simulink model "startOLAE"  (R2021a)
settings: Solver=VariableStepAuto  StartTime=0.0  StopTime=10.0  RelTol=1e-3
libraries: sharedutil x2, dspmtrx3 x1, aerolibutil x1
settings Model: Creator=noraw  LastModifiedBy=noraw

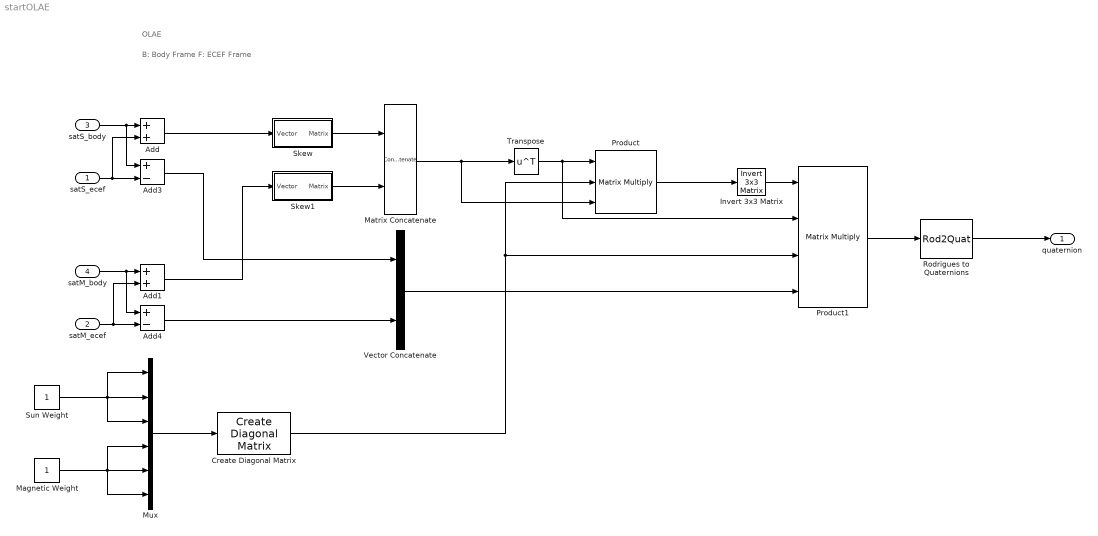
== system startOLAE ==
  note: OLAE
  note: B: Body Frame
      | F: ECEF Frame
  satS_ecef : Inport  PortDimensions=3
  satM_ecef : Inport  Port=2  PortDimensions=3
  satS_body : Inport  Port=3  PortDimensions=3
  satM_body : Inport  Port=4  PortDimensions=3
  Add : Sum
  Add1 : Sum
  Add3 : Sum  Inputs=+-
  Add4 : Sum  Inputs=+-
  Create Diagonal Matrix : dspmtrx3/Create Diagonal Matrix
      settings: SourceProductBaseCode=DS
  Invert 3x3 Matrix : aerolibutil/Invert  3x3 Matrix
  Magnetic Weight : Constant
  Matrix Concatenate : Concatenate  Mode=Multidimensional array
  Mux : Mux  Inputs=6
  Product : Product  Inputs=3  Multiplication=Matrix(*)
  Product1 : Product  Inputs=4  Multiplication=Matrix(*)
  Rodrigues to Quaternions : Rod2Quat
  Skew : Subsystem
  Skew1 : Subsystem
  Sun Weight : Constant
  Transpose : Math  Operator=transpose  SaturateOnIntegerOverflow=on
  Vector Concatenate : Concatenate
  quaternion : Outport
  wires:
  Matrix Concatenate/1 -> Product/3, Transpose/1
  Product/1 -> Invert 3x3 Matrix/1
  Sun Weight/1 -> Mux/1, Mux/2, Mux/3
  Invert 3x3 Matrix/1 -> Product1/1
  Product1/1 -> Rodrigues to Quaternions/1
  Transpose/1 -> Product1/2, Product/1
  Skew/1(Matrix) -> Matrix Concatenate/1
  Magnetic Weight/1 -> Mux/4, Mux/5, Mux/6
  Skew1/1(Matrix) -> Matrix Concatenate/2
  Create Diagonal Matrix/1 -> Product/2, Product1/3
  Mux/1 -> Create Diagonal Matrix/1
  satS_body/1 -> Add3/1, Add/1
  Add1/1 -> Skew1/1(Vector)
  satM_ecef/1 -> Add1/2, Add4/2
  Add/1 -> Skew/1(Vector)
  satM_body/1 -> Add4/1, Add1/1
  Add4/1 -> Vector Concatenate/2
  Rodrigues to Quaternions/1 -> quaternion/1
  Add3/1 -> Vector Concatenate/1
  satS_ecef/1 -> Add/2, Add3/2
  Vector Concatenate/1 -> Product1/4

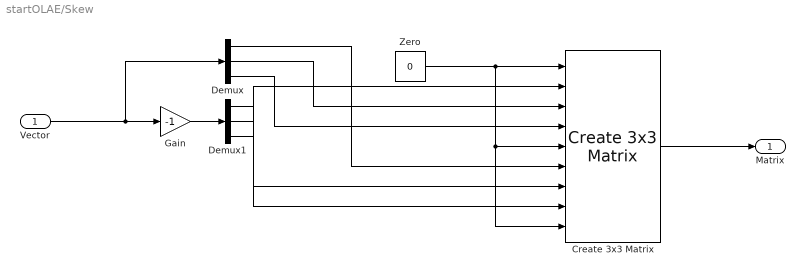
== system startOLAE/Skew ==
  Vector : Inport
  Create 3x3 Matrix : sharedutil/Create 3x3 Matrix  aMode=aMode
      settings: SourceProductBaseCode=AE,PW,MT,UV,VE,VP
  Demux : Demux  Outputs=3
  Demux1 : Demux  Outputs=3
  Gain : Gain  Gain=-1
  Zero : Constant  Value=0  OutDataTypeStr=Inherit: Inherit via back propagation
  Matrix : Outport
  wires:
  Gain/1 -> Demux1/1
  Demux/1 -> Create 3x3 Matrix/6
  Demux1/2 -> Create 3x3 Matrix/7
  Vector/1 -> Gain/1, Demux/1
  Demux1/1 -> Create 3x3 Matrix/8
  Demux1/3 -> Create 3x3 Matrix/2
  Zero/1 -> Create 3x3 Matrix/9, Create 3x3 Matrix/5, Create 3x3 Matrix/1
  Demux/3 -> Create 3x3 Matrix/4
  Demux/2 -> Create 3x3 Matrix/3
  Create 3x3 Matrix/1 -> Matrix/1

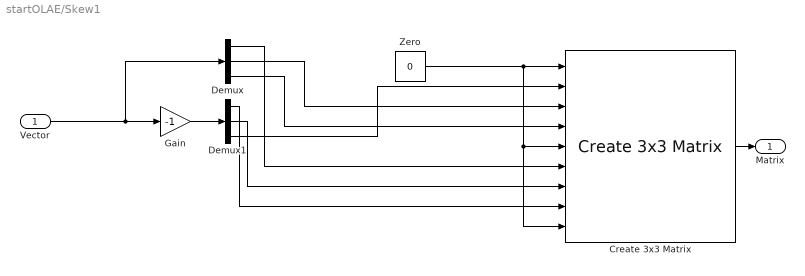
== system startOLAE/Skew1 ==
  Vector : Inport
  Create 3x3 Matrix : sharedutil/Create 3x3 Matrix  aMode=aMode
      settings: SourceProductBaseCode=AE,PW,MT,UV,VE,VP
  Demux : Demux  Outputs=3
  Demux1 : Demux  Outputs=3
  Gain : Gain  Gain=-1
  Zero : Constant  Value=0  OutDataTypeStr=Inherit: Inherit via back propagation
  Matrix : Outport
  wires:
  Gain/1 -> Demux1/1
  Demux/1 -> Create 3x3 Matrix/6
  Demux1/2 -> Create 3x3 Matrix/7
  Vector/1 -> Gain/1, Demux/1
  Demux1/1 -> Create 3x3 Matrix/8
  Demux1/3 -> Create 3x3 Matrix/2
  Zero/1 -> Create 3x3 Matrix/9, Create 3x3 Matrix/5, Create 3x3 Matrix/1
  Demux/3 -> Create 3x3 Matrix/4
  Demux/2 -> Create 3x3 Matrix/3
  Create 3x3 Matrix/1 -> Matrix/1
